simulink model "OTDOA_Positioning_Model2"  (R2023b)
settings: Solver=VariableStepAuto  StartTime=0.0  StopTime=10.0  RelTol=1e-3
undefined symbols (not defined in the file or in its folder): phased, physconst
libraries: phasedtxrxlib x6, commchan3 x3, commrflib2 x3
settings Model: Creator=Talha  LastModifiedBy=Oluwaseun

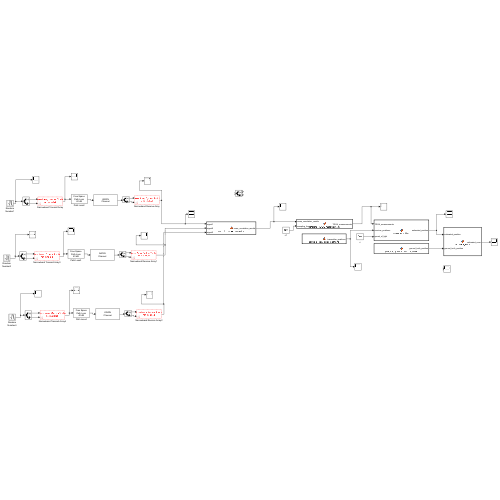
[thumbnail: Simulink's stored preview of the top-level diagram]
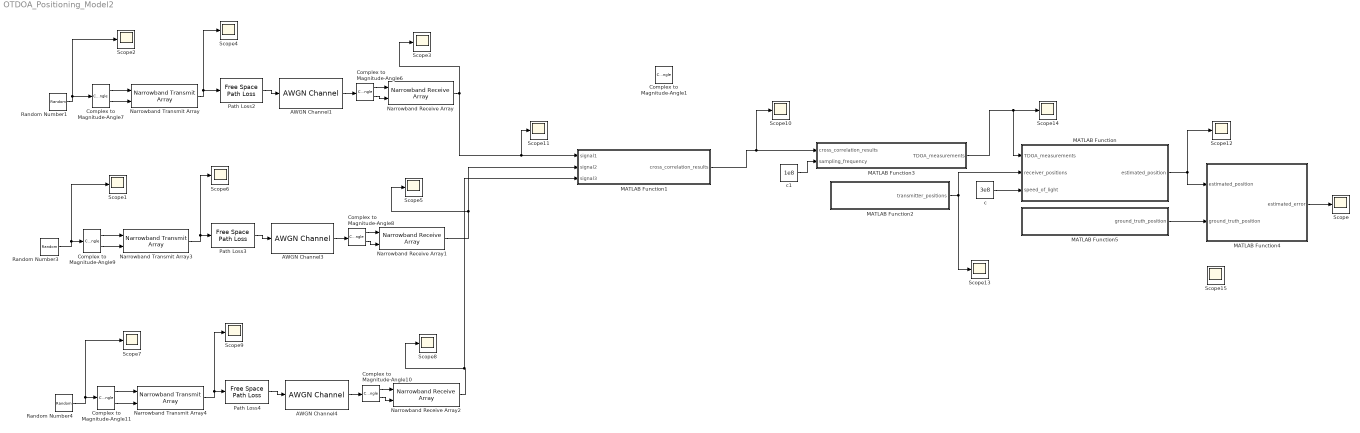
== system OTDOA_Positioning_Model2 ==
  AWGN Channel1 : commchan3/AWGN Channel  LegacyMode=off  NoiseMethod="Signal to noise ratio  (SNR)"  noiseMode="Signal to noise ratio  (SNR)"  EbNo=10  EsNo=10  SNR=20  BitsPerSymbol=1  SignalPower=1e-9  SamplesPerSymbol=1  SymbolPeriod=1  VarianceSource=Parameter  Variance=1  RandomStream=Global stream  Seed=67  SimulateUsing=Code generation
  AWGN Channel3 : commchan3/AWGN Channel  LegacyMode=off  NoiseMethod="Signal to noise ratio  (SNR)"  noiseMode="Signal to noise ratio  (SNR)"  EbNo=10  EsNo=10  SNR=20  BitsPerSymbol=1  SignalPower=1e-9  SamplesPerSymbol=1  SymbolPeriod=1  VarianceSource=Parameter  Variance=1  RandomStream=Global stream  Seed=67  SimulateUsing=Code generation
  AWGN Channel4 : commchan3/AWGN Channel  LegacyMode=off  NoiseMethod="Signal to noise ratio  (SNR)"  noiseMode="Signal to noise ratio  (SNR)"  EbNo=10  EsNo=10  SNR=20  BitsPerSymbol=1  SignalPower=1e-9  SamplesPerSymbol=1  SymbolPeriod=1  VarianceSource=Parameter  Variance=1  RandomStream=Global stream  Seed=67  SimulateUsing=Code generation
  Complex to Magnitude-Angle{1,6..11} (7 alike) : ComplexToMagnitudeAngle
  MATLAB Function : MATLAB Function  TreatAsAtomicUnit=on
  MATLAB Function1 : MATLAB Function  TreatAsAtomicUnit=on
  MATLAB Function2 : MATLAB Function  TreatAsAtomicUnit=on
  MATLAB Function3 : MATLAB Function  TreatAsAtomicUnit=on
  MATLAB Function4 : MATLAB Function  TreatAsAtomicUnit=on
  MATLAB Function5 : MATLAB Function  TreatAsAtomicUnit=on
  Narrowband Receive Array : phasedtxrxlib/Narrowband Receive Array  PropagationSpeed=physconst( 'LightSpeed' )  OperatingFrequency=3e8  Wavefront=Plane  SensorGainMeasure=dB  Polarization=None  WeightsInputPort=off  SimulateUsing=Interpreted execution  Sensor=phased.OmnidirectionalMicrophoneElement()
  Narrowband Receive Array1 : phasedtxrxlib/Narrowband Receive Array  PropagationSpeed=physconst( 'LightSpeed' )  OperatingFrequency=3e8  Wavefront=Plane  SensorGainMeasure=dB  Polarization=None  WeightsInputPort=off  SimulateUsing=Interpreted execution  Sensor=phased.OmnidirectionalMicrophoneElement()
  Narrowband Receive Array2 : phasedtxrxlib/Narrowband Receive Array  PropagationSpeed=physconst( 'LightSpeed' )  OperatingFrequency=3e8  Wavefront=Plane  SensorGainMeasure=dB  Polarization=None  WeightsInputPort=off  SimulateUsing=Interpreted execution  Sensor=phased.OmnidirectionalMicrophoneElement()
  Narrowband Transmit Array : phasedtxrxlib/Narrowband Transmit Array  PropagationSpeed=physconst( 'LightSpeed' )  OperatingFrequency=3e8  CombineRadiatedSignals=on  SensorGainMeasure=dB  Polarization=None  WeightsInputPort=off  SimulateUsing=Interpreted execution  Sensor=phased.OmnidirectionalMicrophoneElement()
  Narrowband Transmit Array3 : phasedtxrxlib/Narrowband Transmit Array  PropagationSpeed=physconst( 'LightSpeed' )  OperatingFrequency=3e8  CombineRadiatedSignals=on  SensorGainMeasure=dB  Polarization=None  WeightsInputPort=off  SimulateUsing=Interpreted execution  Sensor=phased.OmnidirectionalMicrophoneElement()
  Narrowband Transmit Array4 : phasedtxrxlib/Narrowband Transmit Array  PropagationSpeed=physconst( 'LightSpeed' )  OperatingFrequency=3e8  CombineRadiatedSignals=on  SensorGainMeasure=dB  Polarization=None  WeightsInputPort=off  SimulateUsing=Interpreted execution  Sensor=phased.OmnidirectionalMicrophoneElement()
  Path Loss2 : commrflib2/Free Space Path Loss  mode=Decibels  dB=40  d=0.100  fc=1920
  Path Loss3 : commrflib2/Free Space Path Loss  mode=Decibels  dB=40  d=0.100  fc=1920
  Path Loss4 : commrflib2/Free Space Path Loss  mode=Decibels  dB=40  d=0.100  fc=1920
  Random Number1 : RandomNumber  Mean=-70  Variance=10  SampleTime=1  VectorParams1D=off
  Random Number3 : RandomNumber  Mean=-70  Variance=10  SampleTime=1  VectorParams1D=off
  Random Number4 : RandomNumber  Mean=-70  Variance=10  SampleTime=1  VectorParams1D=off
  Scope{,1..15} (16 alike) : Scope
  c : Constant  Value=3e8
  c1 : Constant  Value=1e8
  wires:
  MATLAB Function2/1(transmitter_positions) -> Scope13/1, MATLAB Function/2(receiver_positions)
  c/1 -> MATLAB Function/3(speed_of_light)
  MATLAB Function4/1(estimated_error) -> Scope/1
  MATLAB Function5/1(ground_truth_position) -> MATLAB Function4/2(ground_truth_position)
  c1/1 -> MATLAB Function3/2(sampling_frequency)
  Complex to Magnitude-Angle7/2 -> Narrowband Transmit Array/2
  Complex to Magnitude-Angle7/1 -> Narrowband Transmit Array/1
  Random Number1/1 -> Scope2/1, Complex to Magnitude-Angle7/1
  Complex to Magnitude-Angle6/2 -> Narrowband Receive Array/2
  Complex to Magnitude-Angle6/1 -> Narrowband Receive Array/1
  Narrowband Transmit Array/1 -> Scope4/1, Path Loss2/1
  AWGN Channel1/1 -> Complex to Magnitude-Angle6/1
  Path Loss2/1 -> AWGN Channel1/1
  Complex to Magnitude-Angle9/1 -> Narrowband Transmit Array3/1
  Narrowband Transmit Array3/1 -> Scope6/1, Path Loss3/1
  Complex to Magnitude-Angle8/2 -> Narrowband Receive Array1/2
  Random Number3/1 -> Scope1/1, Complex to Magnitude-Angle9/1
  Path Loss3/1 -> AWGN Channel3/1
  Complex to Magnitude-Angle9/2 -> Narrowband Transmit Array3/2
  AWGN Channel3/1 -> Complex to Magnitude-Angle8/1
  Complex to Magnitude-Angle8/1 -> Narrowband Receive Array1/1
  Complex to Magnitude-Angle11/1 -> Narrowband Transmit Array4/1
  Narrowband Transmit Array4/1 -> Scope9/1, Path Loss4/1
  Complex to Magnitude-Angle10/2 -> Narrowband Receive Array2/2
  Random Number4/1 -> Scope7/1, Complex to Magnitude-Angle11/1
  Path Loss4/1 -> AWGN Channel4/1
  Complex to Magnitude-Angle11/2 -> Narrowband Transmit Array4/2
  AWGN Channel4/1 -> Complex to Magnitude-Angle10/1
  Complex to Magnitude-Angle10/1 -> Narrowband Receive Array2/1
  MATLAB Function1/1(cross_correlation_results) -> MATLAB Function3/1(cross_correlation_results), Scope10/1
  Narrowband Receive Array2/1 -> MATLAB Function1/3(signal3), Scope8/1
  Narrowband Receive Array/1 -> Scope11/1, MATLAB Function1/1(signal1), Scope3/1
  Narrowband Receive Array1/1 -> MATLAB Function1/2(signal2), Scope5/1
  MATLAB Function3/1(TDOA_measurements) -> Scope14/1, MATLAB Function/1(TDOA_measurements)
  MATLAB Function/1(estimated_position) -> MATLAB Function4/1(estimated_position), Scope12/1

== matlab function OTDOA_Positioning_Model2/MATLAB Function1 ==
  data: signal1 input; cross_correlation_results output; signal2 input; signal3 input
function cross_correlation_results = compute_cross_correlation(signal1, signal2, signal3)
    % Check if input signals are continuous series
    if ~isvector(signal1) || ~isvector(signal2) || ~isvector(signal3)
        error('Input signals must be vectors representing continuous series.');
    end
    
    % Compute cross-correlation between signals received by three receivers
    
    % Compute cross-correlation between signal1 and signal2
    cross_corr_12 = sum(signal1 .* signal2);
    
    % Compute cross-correlation between signal1 and signal3
    cross_corr_13 = sum(signal1 .* signal3);
    
    % Compute cross-correlation between signal2 and signal3
    cross_corr_23 = sum(signal2 .* signal3);
    
    % Combine cross-correlation results
    cross_correlation_results = [cross_corr_12, cross_corr_13, cross_corr_23];
end

== matlab function OTDOA_Positioning_Model2/MATLAB Function ==
  data: TDOA_measurements input; estimated_position output; receiver_positions input; speed_of_light input
function estimated_position = otdoa_algorithm(TDOA_measurements, receiver_positions, speed_of_light)
    % Check if input TDOA_measurements is a vector
    if ~isvector(TDOA_measurements)
        error('TDOA measurements must be a vector.');
    end
    
    % Number of receivers
    num_receivers = size(receiver_positions, 1);

    % Initialize estimated position
    estimated_position = zeros(1, 2); % Adjusted for 2D positions

    % Check if TDOA_measurements has at least two elements
    if numel(TDOA_measurements) >= 2
        % Initialize accumulator for estimated positions
        accumulated_position = zeros(1, 2);

        % Iterate through receiver pairs to find intersection points
        for i = 1:num_receivers-1
            for j = i+1:num_receivers
                % Calculate distance difference between receiver pairs
                delta_dist = (TDOA_measurements(j) - TDOA_measurements(i)) * speed_of_light;

                % Calculate vector between receiver positions
                vec_ij = receiver_positions(j, :) - receiver_positions(i, :);
                dist_ij = norm(vec_ij);
                
                % Check if the distance between receivers is not too small
                if dist_ij > 0.001 % Adjust this threshold as needed
                    % Calculate unit vector
                    unit_vec_ij = vec_ij / dist_ij;

                    % Calculate intersection point
                    intersection_point = receiver_positions(i, :) + (delta_dist / 2) * unit_vec_ij;

                    % Accumulate intersection points
                    accumulated_position = accumulated_position + intersection_point;
                end
            end
        end

        % Calculate average estimated position
        estimated_position = accumulated_position / (num_receivers * (num_receivers - 1) / 2);
    else
        % Return the estimated position based on the single TDOA measurement
        estimated_position = receiver_positions(1, :);
    end
end

== matlab function OTDOA_Positioning_Model2/MATLAB Function2 ==
  data: transmitter_positions output
function transmitter_positions = calculate_transmitter_positions()
    % Define transmitter positions
    transmitter1_position = [1, 1];  % Transmitter 1 position (x, y) in meters
    transmitter2_position = [5, 1];  % Transmitter 2 position (x, y) in meters
    transmitter3_position = [1, 5];  % Transmitter 3 position (x, y) in meters
    
    % Store transmitter positions in a matrix
    transmitter_positions = [transmitter1_position; transmitter2_position; transmitter3_position];
    
    % Check if any transmitter position is [0, 0]
    if any(all(transmitter_positions == 0, 2))
        error('Error: Transmitter positions include a flat 0 line.');
    end
end

== matlab function OTDOA_Positioning_Model2/MATLAB Function3 ==
  data: cross_correlation_results input; TDOA_measurements output; sampling_frequency input
function TDOA_measurements = generate_TDOA_measurements(cross_correlation_results, sampling_frequency)
    % Check if input cross-correlation results is a vector
    if ~isvector(cross_correlation_results)
        error('Cross-correlation results must be a vector.');
    end
    
    % Find the peak index in the cross-correlation results
    [~, peak_index] = max(cross_correlation_results);

    % Calculate TDOA measurements based on the peak index and sampling frequency
    TDOA_measurements = peak_index / sampling_frequency;
end

== matlab function OTDOA_Positioning_Model2/MATLAB Function4 ==
  data: estimated_position input; estimated_error output; ground_truth_position input
function estimated_error = calculate_error(estimated_position, ground_truth_position)
    % Check if inputs are row vectors of the same length
    if ~isvector(estimated_position) || ~isvector(ground_truth_position) || numel(estimated_position) ~= numel(ground_truth_position)
        error('Input positions must be row vectors of the same length.');
    end
    
    % Calculate the error between estimated position and ground truth position
    % Compute error vector
    error_vector = estimated_position - ground_truth_position;
    
    % Calculate Euclidean distance (magnitude) of the error vector
    estimated_error = norm(error_vector);
end

== matlab function OTDOA_Positioning_Model2/MATLAB Function5 ==
  data: ground_truth_position output
function ground_truth_position = generate_ground_truth_position()
    % Generate ground truth position
    
    % Example: Generating random x and y coordinates within a predefined range
    min_range = -100; % Minimum value for position coordinates
    max_range = 100;  % Maximum value for position coordinates
    
    % Generate random x and y coordinates within the range
    x = min_range + (max_range - min_range) * rand();
    y = min_range + (max_range - min_range) * rand();
    
    % Construct ground truth position vector
    ground_truth_position = [x, y];
end
